simulink model "tests"  (R2021b)
settings: Solver=VariableStepAuto  StartTime=0.0  StopTime=0.1  RelTol=1e-3
InitFcn:
  | init_fcn
values from neighbouring files (symbols this model uses):
  Tint = 1e-6    (= 1e-06)    [init_fcn.m]
libraries: spsCurrentMeasurementLib x3, spsVoltageMeasurementLib x3, spsThreePhaseSeriesRLCLoadLib x1, spsThreePhaseSourceLib x1, spspowerguiLib x1
settings Model: Creator=david  LastModifiedBy=david

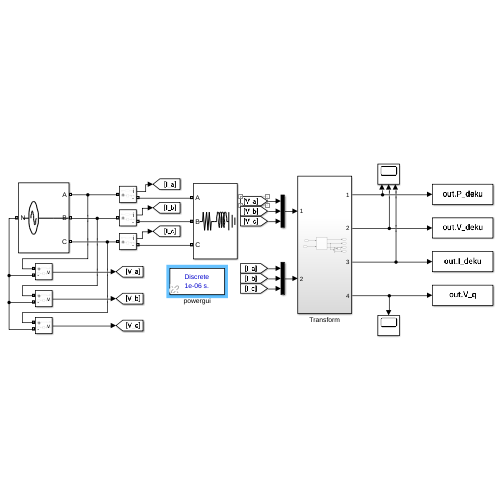
[thumbnail: Simulink's stored preview of the top-level diagram]
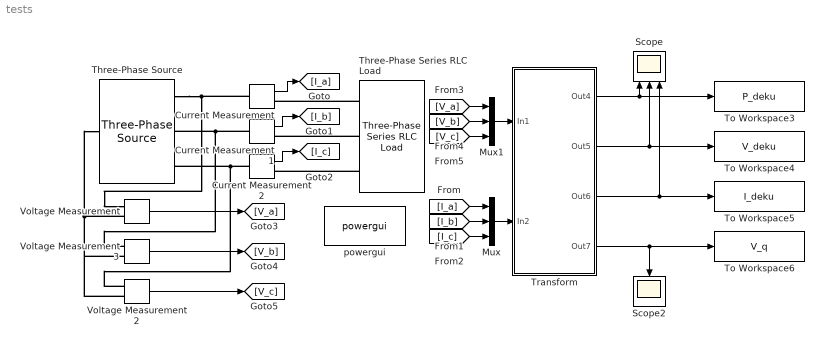
== system tests ==
  Current Measurement : spsCurrentMeasurementLib/Current Measurement  PhasorSimulation=off  OutputType=Complex  PSBequivalent=0
  Current Measurement1 : spsCurrentMeasurementLib/Current Measurement  PhasorSimulation=off  OutputType=Complex  PSBequivalent=0
  Current Measurement2 : spsCurrentMeasurementLib/Current Measurement  PhasorSimulation=off  OutputType=Complex  PSBequivalent=0
  Mux : Mux  Inputs=3
  Mux1 : Mux  Inputs=3
  Scope : Scope  NumInputPorts=3
  Scope2 : Scope
  Three-Phase Series RLC Load : spsThreePhaseSeriesRLCLoadLib/Three-Phase Series RLC Load  LConnTagsString=A|B|C  Configuration=Y (grounded)  NominalVoltage=400  Vabc=[1e3 1e3 1e3]  Vabcp=[1e3 1e3 1e3]  NominalFrequency=50  UnbalancedPower=off  ActivePower=10e3  InductivePower=4e3  CapacitivePower=0  Pabc=[10e3 9e3 11e3]  QLabc=[100 90 110]  QCabc=[100 90 110]  Pabcp=[10e3 9e3 11e3]  QLabcp=[100 90 110]  QCabcp=[100 90 110]  Measurements=None  LoadType=constant Z
  Three-Phase Source : spsThreePhaseSourceLib/Three-Phase Source  InternalConnection=Yn  VoltagePhases=off  Voltage=400  PhaseAngle=0  Voltage_phases=[25e3 25e3 25e3]/sqrt(3)  PhaseAngles_phases=[0 -120 +120]  Frequency=50  NonIdealSource=on  SpecifyImpedance=off  Resistance=0  Inductance=0  ShortCircuitLevel=100e6  BaseVoltage=400  XRratio=7  BusType=swing  Pref=10e3  Qref=0  Prefabc=[10e3, 10e3, 10e3]  Qrefabc=[0, 0, 0]  Qmin=-inf  Qmax=inf
  To Workspace3 : ToWorkspace  VariableName=P_deku  SaveFormat=Structure With Time  SampleTime=-1
  To Workspace4 : ToWorkspace  VariableName=V_deku  SaveFormat=Structure With Time  SampleTime=-1
  To Workspace5 : ToWorkspace  VariableName=I_deku  SaveFormat=Structure With Time  SampleTime=-1
  To Workspace6 : ToWorkspace  VariableName=V_q  SaveFormat=Structure With Time  SampleTime=-1
  Transform : Subsystem
  Voltage Measurement : spsVoltageMeasurementLib/Voltage Measurement  PhasorSimulation=off  OutputType=Complex  PSBequivalent=0
  Voltage Measurement2 : spsVoltageMeasurementLib/Voltage Measurement  PhasorSimulation=off  OutputType=Complex  PSBequivalent=0
  Voltage Measurement3 : spsVoltageMeasurementLib/Voltage Measurement  PhasorSimulation=off  OutputType=Complex  PSBequivalent=0
  powergui : spspowerguiLib/powergui  Priority=1  SimulationMode=Discrete  SampleTime=Tint  frequency=60  Iterations=50  frequencyindice=50  Pbase=100e6  ErrMax=1e-4  UnitsV=kV  UnitsW=MW  buscounter=0  FunctionMessages=off  echomessages=off  EnableUseOfTLC=off  CurrentSourceSwitches=off  DisableSnubberDevices=off  DisableRonSwitches=off  DisableVfSwitches=off  DisplayEquations=off  AutomaticDiscreteSolvers=off  SolverType=Tustin/Backward Euler (TBE)  Interpol=off  ExternalGateDelay=off  methode=off  Ts=100  x0status=blocks  SPID=on  SwTol=0  HookPort=off  NonlinearTolerance=1e-4  nMaxIteration=100  ContinueOnMaxIteration=off  RestoreLinks=warning  ResistiveCurrentMeasurement=off  Frange=[0:2:500]  Ylog=off  Xlog=on  ShowGrid=off  save=off  variable=ZData  structure=0  ZoomFFT=off  StartTime=0.0  cycles=1  DisplayStyle=1  fundamental=60  FreqAxis=off  MaxFrequency=1000  frequencyindicesteady=1  RmsSteady=1  display=off
  wires:
  Current Measurement/1 -> [I_a]
  Current Measurement1/1 -> [I_b]
  Current Measurement2/1 -> [I_c]
  Voltage Measurement/1 -> [V_a]
  [I_b] -> Mux/2
  [I_a] -> Mux/1
  [I_c] -> Mux/3
  [V_a] -> Mux1/1
  [V_b] -> Mux1/2
  [V_c] -> Mux1/3
  Voltage Measurement3/1 -> [V_b]
  Voltage Measurement2/1 -> [V_c]
  Mux1/1 -> Transform/1(In1)
  Mux/1 -> Transform/2(In2)
  Transform/1(Out4) -> To Workspace3/1, Scope/1
  Transform/2(Out5) -> To Workspace4/1, Scope/2
  Transform/3(Out6) -> To Workspace5/1, Scope/3
  Transform/4(Out7) -> To Workspace6/1, Scope2/1
  connections:
  Three-Phase Series RLC Load/LConn1 -- Current Measurement/RConn1
  Three-Phase Series RLC Load/LConn2 -- Current Measurement1/RConn1
  Three-Phase Series RLC Load/LConn3 -- Current Measurement2/RConn1
  Three-Phase Source/RConn1 -- Current Measurement/LConn1 -- Voltage Measurement/LConn1
  Current Measurement1/LConn1 -- Voltage Measurement3/LConn1 -- Three-Phase Source/RConn2
  Current Measurement2/LConn1 -- Voltage Measurement2/LConn1 -- Three-Phase Source/RConn3
  Voltage Measurement/LConn2 -- Voltage Measurement3/LConn2 -- Voltage Measurement2/LConn2 -- Three-Phase Source/LConn1

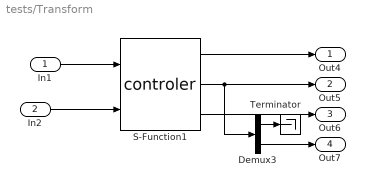
== system tests/Transform ==
  In1 : Inport
  In2 : Inport  Port=2
  Demux3 : Demux  Outputs=2
  S-Function1 : S-Function  FunctionName=controler  SFunctionDeploymentMode=off  EnableBusSupport=off
  Terminator : Terminator
  Out4 : Outport
  Out5 : Outport  Port=2
  Out6 : Outport  Port=3
  Out7 : Outport  Port=4
  wires:
  In1/1 -> S-Function1/1
  Demux3/2 -> Out7/1
  S-Function1/3 -> Out6/1
  In2/1 -> S-Function1/2
  Demux3/1 -> Terminator/1
  S-Function1/1 -> Out4/1
  S-Function1/2 -> Out5/1, Demux3/1
